simulink model "Matrix12"  (R2021a)
settings: Solver=VariableStepAuto  StartTime=0.0  StopTime=1  RelTol=1e-3
undefined symbols (not defined in the file): DiscIntNeverNeededParam
libraries: spsDiodeLib x18, spsIGBTLib x18, simulink x6, spsIGBTDiodeLib x6, spsSeriesRLCBranchLib x4, spsThreePhaseVIMeasurementLib x3, spsSaturableTransformerLib x3, spsabctoAlphaBetaZeroLib x2, spsAlphaBetaZerotoabcLib x1, pid_lib x1, spsSecondOrderFilterLib x1, spsThreePhaseSeriesRLCBranchLib x1
(part 1 of 2)
settings Model: SimulationMode=accelerator  Creator=HP  LastModifiedBy=HP

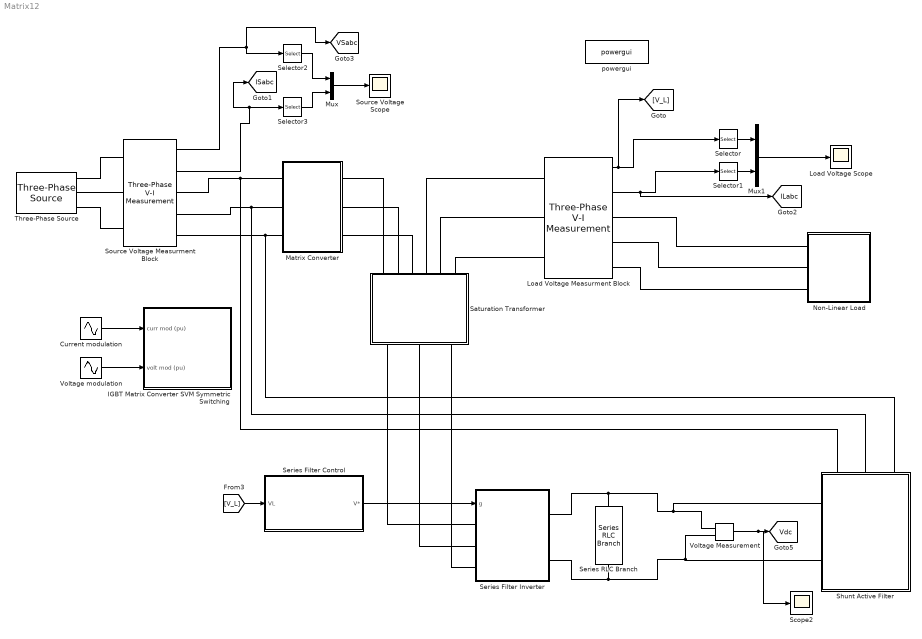
== system Matrix12 ==
  Current modulation : Sin  Amplitude=1*sqrt(2)/sqrt(3)  Frequency=2*pi*1000  Phase=[0 -2*pi/3 2*pi/3]  SampleTime=0
  IGBT Matrix Converter SVM Symmetric Switching : Subsystem
  Load Voltage Measurment Block : spsThreePhaseVIMeasurementLib/Three-Phase V-I Measurement  VoltageMeasurement=phase-to-phase  SetLabelV=off  LabelV=V_L  Vpu=off  VpuLL=off  CurrentMeasurement=yes  SetLabelI=off  LabelI=Iabc  Ipu=off  Pbase=100e6  Vbase=500e3  OutputType=Complex  PhasorSimulation=off  PSBequivalent=0
  Load Voltage Scope : Scope
  Matrix Converter : Subsystem
  Mux : Mux  Inputs=2
  Mux1 : Mux  Inputs=2
  Non-Linear Load : Subsystem
  Saturation Transformer : Subsystem
  Scope2 : Scope
  Selector{,1..3} (4 alike) : Selector  InputPortWidth=3  IndexOptions=Index vector (dialog)  Indices=1  OutputSizes=1
  Series Filter Inverter : Subsystem
      mask Display: fprintf('series\nfilter')
  Series Filter Control : Subsystem
      mask Display: fprintf('Series\nFilter')
  Series RLC Branch : spsSeriesRLCBranchLib/Series RLC Branch  LConnTagsString=__new0  RConnTagsString=__new0  BranchType=C  Resistance=1  Inductance=1e-3  SetiL0=off  InitialCurrent=0  Capacitance=10  Setx0=on  InitialVoltage=700  Measurements=None
  Shunt Active Filter : Subsystem
      settings: PortSchema="{\"entries\":[{\"content\":{\"sides\":[{\"content\":{\"connectorIds\":[]},\"type\":\"ConnectorPlacement.EquallySpacedRectSide\",\"uuid\":\"661bd002-34f2-471b-8915-a7d9af4edb84\"},{\"content\":{\"connectorIds\":[\"RConn1\",\"RConn2\"],\"side\":\"RIGHT\"},\"type\":\"ConnectorPlacement.EquallySpacedRectSide\",\"uuid\":\"4a3a3177-9c19-4181-9982-d76e774c7df0\"},{\"content\":{\"connectorIds\":[\"LConn1\",\"LConn2\",\"LConn3\"],\"side\":\"TOP\"},\"type\":\"ConnectorPlacement.EquallySpacedRectSide\",\"uuid\":\"acd6b456-b827-42fc-a7ca-c38254438ca2\"}]},\"type\":\"ConnectorPlacement.EquallySpacedConnector\",\"uuid\":\"b55db1d3-6588-49b1-b57b-fb04199798b7\"}],\"packageUris\":[\"http://schema.mathworks.com/mf0/Connector/R2020b\"],\"version\":\"1.0\"}"
  Source Voltage Measurment Block : spsThreePhaseVIMeasurementLib/Three-Phase V-I Measurement  VoltageMeasurement=phase-to-ground  SetLabelV=off  LabelV=Vabc  Vpu=off  VpuLL=off  CurrentMeasurement=yes  SetLabelI=off  LabelI=Iabc  Ipu=off  Pbase=100e6  Vbase=500e3  OutputType=Complex  PhasorSimulation=off  PSBequivalent=0
  Source Voltage Scope : Scope
  Three-Phase Source : spsThreePhaseSourceLib/Three-Phase Source  InternalConnection=Yg  VoltagePhases=on  Voltage=400  PhaseAngle=0  Voltage_phases=[400 400 400]/sqrt(3)  PhaseAngles_phases=[0 -120 +120]  Frequency=50  NonIdealSource=off  SpecifyImpedance=off  Resistance=0.8929  Inductance=16.58e-3  ShortCircuitLevel=100e6  BaseVoltage=25e3  XRratio=7  BusType=swing  Pref=10e3  Qref=0  Prefabc=[10e3, 10e3, 10e3]  Qrefabc=[0, 0, 0]  Qmin=-inf  Qmax=inf
  Voltage Measurement : spsVoltageMeasurementLib/Voltage Measurement  PhasorSimulation=off  OutputType=Complex  PSBequivalent=0
  Voltage modulation : Sin  Amplitude=1*sqrt(2)/sqrt(3)  Frequency=2*pi*1000  Phase=[0 -2*pi/3 2*pi/3]  SampleTime=0
  powergui : spspowerguiLib/powergui  SimulationMode=Discrete  SampleTime=2e-6  frequency=50  Iterations=50  frequencyindice=50  Pbase=100e6  ErrMax=1e-4  UnitsV=kV  UnitsW=MW  buscounter=0  FunctionMessages=off  echomessages=off  EnableUseOfTLC=off  CurrentSourceSwitches=off  DisableSnubberDevices=off  DisableRonSwitches=off  DisableVfSwitches=off  DisplayEquations=off  AutomaticDiscreteSolvers=off  SolverType=Tustin/Backward Euler (TBE)  Interpol=off  ExternalGateDelay=off  methode=off  Ts=100  x0status=blocks  SPID=off  SwTol=0  HookPort=off  NonlinearTolerance=1e-4  nMaxIteration=100  ContinueOnMaxIteration=off  RestoreLinks=warning  ResistiveCurrentMeasurement=off  Frange=[0:2:500]  Ylog=off  Xlog=on  ShowGrid=off  save=off  variable=ZData  structure=Vs  ZoomFFT=on  StartTime=1/60  cycles=1  DisplayStyle=1  fundamental=60  FreqAxis=on  MaxFrequency=10000  frequencyindicesteady=1  RmsSteady=1  display=off
  tag scope: ILabc=global, ISabc=global, VSabc=global, Vdc=global
  wires:
  [V_L] -> Series Filter Control/1(VL)
  Mux/1 -> Source Voltage Scope/1
  Selector1/1 -> Mux1/2
  Selector/1 -> Mux1/1
  Load Voltage Measurment Block/1 -> [V_L], Selector/1
  Selector3/1 -> Mux/2
  Source Voltage Measurment Block/1 -> Selector2/1, [VSabc]
  Series Filter Control/1(V*) -> Series Filter Inverter/1(g)
  Source Voltage Measurment Block/2 -> [ISabc], Selector3/1
  Voltage modulation/1 -> IGBT Matrix Converter SVM Symmetric Switching/2(volt mod (pu))
  Load Voltage Measurment Block/2 -> [ILabc], Selector1/1
  Mux1/1 -> Load Voltage Scope/1
  Current modulation/1 -> IGBT Matrix Converter SVM Symmetric Switching/1(curr mod (pu))
  Selector2/1 -> Mux/1
  Voltage Measurement/1 -> Scope2/1, [Vdc]
  connections:
  Series Filter Inverter/LConn3 -- Saturation Transformer/LConn3
  Series Filter Inverter/LConn1 -- Saturation Transformer/LConn1
  Saturation Transformer/RConn3 -- Matrix Converter/RConn3
  Saturation Transformer/RConn4 -- Load Voltage Measurment Block/LConn1
  Source Voltage Measurment Block/RConn2 -- Matrix Converter/LConn2 -- Shunt Active Filter/LConn2
  Saturation Transformer/RConn5 -- Load Voltage Measurment Block/LConn2
  Series Filter Inverter/LConn2 -- Saturation Transformer/LConn2
  Three-Phase Source/RConn1 -- Source Voltage Measurment Block/LConn1
  Source Voltage Measurment Block/RConn3 -- Shunt Active Filter/LConn1 -- Matrix Converter/LConn3
  Three-Phase Source/RConn2 -- Source Voltage Measurment Block/LConn2
  Saturation Transformer/RConn1 -- Matrix Converter/RConn1
  Three-Phase Source/RConn3 -- Source Voltage Measurment Block/LConn3
  Saturation Transformer/RConn2 -- Matrix Converter/RConn2
  Saturation Transformer/RConn6 -- Load Voltage Measurment Block/LConn3
  Matrix Converter/LConn1 -- Shunt Active Filter/LConn3 -- Source Voltage Measurment Block/RConn1
  Voltage Measurement/LConn1 -- Series RLC Branch/LConn1 -- Series Filter Inverter/RConn1 -- Shunt Active Filter/RConn1
  Shunt Active Filter/RConn2 -- Series RLC Branch/RConn1 -- Series Filter Inverter/RConn2 -- Voltage Measurement/LConn2
  Load Voltage Measurment Block/RConn1 -- Non-Linear Load/LConn1
  Load Voltage Measurment Block/RConn2 -- Non-Linear Load/LConn2
  Load Voltage Measurment Block/RConn3 -- Non-Linear Load/LConn3

== system Matrix12/IGBT Matrix Converter SVM Symmetric Switching ==
  curr mod (pu) : Inport
  volt mod (pu) : Inport  Port=2
  SVM Inversion symmetric sequence : Subsystem  mask{switching_freq=1000}
      mask prompts: switching_freq "switching frequency (Hz)"
  SVM Rectification symmetric sequence : Subsystem  mask{switching_freq=1000}
      mask prompts: switching_freq "switching frequency (Hz)"
  matrix converter switching : Subsystem
  wires:
  SVM Inversion symmetric sequence/1(g) -> matrix converter switching/2(gI)
  SVM Rectification symmetric sequence/1(g) -> matrix converter switching/1(gR)
  curr mod (pu)/1 -> SVM Rectification symmetric sequence/1(mod (pu))
  volt mod (pu)/1 -> SVM Inversion symmetric sequence/1(mod (pu))

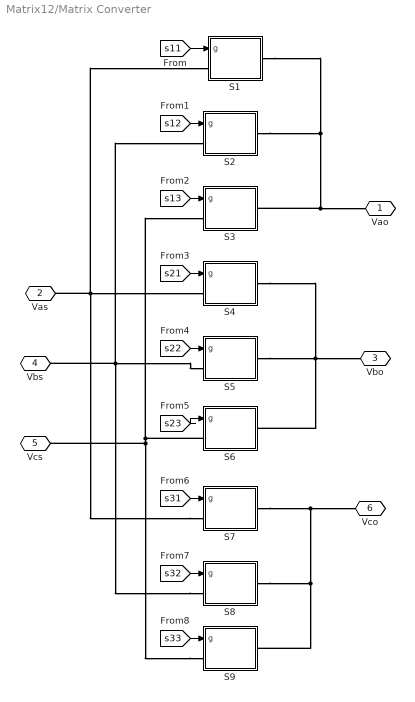
== system Matrix12/Matrix Converter ==
  S1 : Subsystem
  S2 : Subsystem
  S3 : Subsystem
  S4 : Subsystem
  S5 : Subsystem
  S6 : Subsystem
  S7 : Subsystem
  S8 : Subsystem
  S9 : Subsystem
  Vao : PMIOPort  Side=Right
  Vas : PMIOPort  Port=2  Side=Left
  Vbo : PMIOPort  Port=3  Side=Right
  Vbs : PMIOPort  Port=4  Side=Left
  Vcs : PMIOPort  Port=5  Side=Left
  Vco : PMIOPort  Port=6  Side=Right
  wires:
  [s12] -> S2/1(g)
  [s13] -> S3/1(g)
  [s32] -> S8/1(g)
  [s11] -> S1/1(g)
  [s33] -> S9/1(g)
  [s31] -> S7/1(g)
  [s23] -> S6/1(g)
  [s22] -> S5/1(g)
  [s21] -> S4/1(g)
  connections:
  S3/RConn1 -- S1/RConn1 -- S2/RConn1 -- Vao/RConn1
  S7/LConn1 -- S1/LConn1 -- S4/LConn1 -- Vas/RConn1
  S6/RConn1 -- S4/RConn1 -- S5/RConn1 -- Vbo/RConn1
  S8/LConn1 -- S2/LConn1 -- S5/LConn1 -- Vbs/RConn1
  S9/RConn1 -- S8/RConn1 -- S7/RConn1 -- Vco/RConn1
  S9/LConn1 -- S3/LConn1 -- S6/LConn1 -- Vcs/RConn1

== system Matrix12/Non-Linear Load ==
  Series RLC Branch : spsSeriesRLCBranchLib/Series RLC Branch  LConnTagsString=__new0  RConnTagsString=__new0  BranchType=RL  Resistance=10  Inductance=1e-6  SetiL0=off  InitialCurrent=0  Capacitance=1e-6  Setx0=off  InitialVoltage=0  Measurements=None
  Series RLC Branch1 : spsSeriesRLCBranchLib/Series RLC Branch  LConnTagsString=__new0  RConnTagsString=__new0  BranchType=RL  Resistance=10  Inductance=1e-6  SetiL0=off  InitialCurrent=0  Capacitance=1e-6  Setx0=off  InitialVoltage=0  Measurements=None
  Series RLC Branch2 : spsSeriesRLCBranchLib/Series RLC Branch  LConnTagsString=__new0  RConnTagsString=__new0  BranchType=RL  Resistance=10  Inductance=1e-6  SetiL0=off  InitialCurrent=0  Capacitance=1e-6  Setx0=off  InitialVoltage=0  Measurements=None
  a : PMIOPort  Side=Left
  b : PMIOPort  Port=2  Side=Left
  c : PMIOPort  Port=3  Side=Left
  connections:
  a/RConn1 -- Series RLC Branch/LConn1
  Series RLC Branch/RConn1 -- Series RLC Branch1/RConn1 -- Series RLC Branch2/RConn1
  b/RConn1 -- Series RLC Branch1/LConn1
  c/RConn1 -- Series RLC Branch2/LConn1

== system Matrix12/Saturation Transformer ==
  Tc_a : spsSaturableTransformerLib/Saturable Transformer  ThreeWindings=off  Hysteresis=off  DataFile='hysteresis.mat'  Measurements=None  UNITS=pu  NominalPower=[4000 50]  Winding1="[400  0.02  0.02 ]"  Winding2="[400  0.02  0.02]"  Winding3="[ 315e3  0.002  0.08 ]"  Saturation=[ 0 0 ;1.016 9.043]*1e-3  CoreLoss=[117 0]  BreakLoop=off  DiscreteSolver=Trapezoidal iterative  DataType=off  InitialFlux=0  TransfoNumber=1
      settings: SourceProductBaseCode=PS
  Tc_b : spsSaturableTransformerLib/Saturable Transformer  ThreeWindings=off  Hysteresis=off  DataFile='hysteresis.mat'  Measurements=None  UNITS=pu  NominalPower=[4000 50]  Winding1="[400  0.02  0.02 ]"  Winding2="[400  0.02  0.02]"  Winding3="[ 315e3  0.002  0.08 ]"  Saturation=[ 0 0 ;1.016 9.043]*1e-3  CoreLoss=[117 0]  BreakLoop=off  DiscreteSolver=Trapezoidal iterative  DataType=off  InitialFlux=0  TransfoNumber=1
      settings: SourceProductBaseCode=PS
  Tc_c : spsSaturableTransformerLib/Saturable Transformer  ThreeWindings=off  Hysteresis=off  DataFile='hysteresis.mat'  Measurements=None  UNITS=pu  NominalPower=[4000 50]  Winding1="[400  0.02  0.02 ]"  Winding2="[400  0.02  0.02]"  Winding3="[ 315e3  0.002  0.08 ]"  Saturation=[ 0 0 ;1.016 9.043]*1e-3  CoreLoss=[117 0]  BreakLoop=off  DiscreteSolver=Trapezoidal iterative  DataType=off  InitialFlux=0  TransfoNumber=1
      settings: SourceProductBaseCode=PS
  A : PMIOPort  Side=Left
  B : PMIOPort  Port=2  Side=Left
  C : PMIOPort  Port=3  Side=Left
  Vain : PMIOPort  Port=4  Side=Right
  Vbin : PMIOPort  Port=5  Side=Right
  Vcin : PMIOPort  Port=6  Side=Right
  Vao : PMIOPort  Port=7  Side=Right
  Vbo : PMIOPort  Port=8  Side=Right
  Vco : PMIOPort  Port=9  Side=Right
  connections:
  Tc_c/LConn2 -- C/RConn1
  Tc_a/RConn2 -- Vao/RConn1
  Vcin/RConn1 -- Tc_c/RConn1
  Tc_a/LConn1 -- Tc_c/LConn1 -- Tc_b/LConn1
  Tc_b/LConn2 -- B/RConn1
  Vain/RConn1 -- Tc_a/RConn1
  Tc_c/RConn2 -- Vco/RConn1
  Vbin/RConn1 -- Tc_b/RConn1
  Tc_b/RConn2 -- Vbo/RConn1
  Tc_a/LConn2 -- A/RConn1

== system Matrix12/Series Filter Inverter ==
  g : Inport
  Demux : Demux  Outputs=3
      settings: DisplayOption=none
  Logical Operator : Logic  Operator=NOT  AllPortsSameDT=off  OutDataTypeStr=boolean
  Logical Operator1 : Logic  Operator=NOT  AllPortsSameDT=off  OutDataTypeStr=boolean
  Logical Operator2 : Logic  Operator=NOT  AllPortsSameDT=off  OutDataTypeStr=boolean
  s{1..6} (6 alike) : spsIGBTDiodeLib/IGBT//Diode  Ron=1e-3  Rs=1e5  Cs=inf  Measurements=off
  + : PMIOPort  Side=Right
  - : PMIOPort  Port=2  Side=Right
  A : PMIOPort  Port=3  Side=Left
  B : PMIOPort  Port=4  Side=Left
  C : PMIOPort  Port=5  Side=Left
  wires:
  Demux/2 -> s3/1, Logical Operator1/1
  Demux/1 -> s1/1, Logical Operator/1
  Logical Operator/1 -> s2/1
  Logical Operator1/1 -> s4/1
  Logical Operator2/1 -> s6/1
  Demux/3 -> Logical Operator2/1, s5/1
  g/1 -> Demux/1
  connections:
  +/RConn1 -- s5/LConn1 -- s1/LConn1 -- s3/LConn1
  A/RConn1 -- s2/LConn1 -- s1/RConn1
  -/RConn1 -- s6/RConn1 -- s4/RConn1 -- s2/RConn1
  B/RConn1 -- s4/LConn1 -- s3/RConn1
  C/RConn1 -- s5/RConn1 -- s6/LConn1

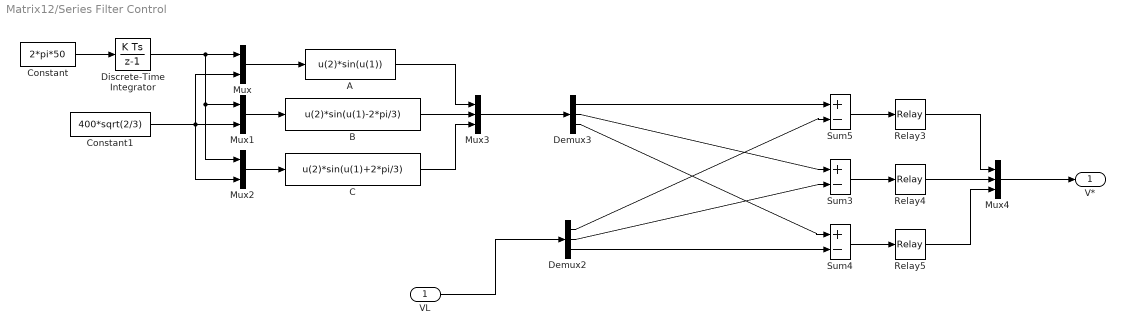
== system Matrix12/Series Filter Control ==
  VL : Inport
  A : Fcn  Expr=u(2)*sin(u(1))
  B : Fcn  Expr=u(2)*sin(u(1)-2*pi/3)
  C : Fcn  Expr=u(2)*sin(u(1)+2*pi/3)
  Constant : Constant  Value=2*pi*50
  Constant1 : Constant  Value=400*sqrt(2/3)
  Demux2 : Demux  Outputs=3
  Demux3 : Demux  Outputs=3
  Discrete-Time Integrator : DiscreteIntegrator  SampleTime=2e-6  ICPrevOutput=DiscIntNeverNeededParam  ICPrevScaledInput=DiscIntNeverNeededParam
  Mux : Mux  Inputs=2
  Mux1 : Mux  Inputs=2
  Mux2 : Mux  Inputs=2
  Mux3 : Mux  Inputs=3
  Mux4 : Mux  Inputs=3
  Relay3 : Relay  OnSwitchValue=1  OffSwitchValue=-1
  Relay4 : Relay  OnSwitchValue=1  OffSwitchValue=-1
  Relay5 : Relay  OnSwitchValue=1  OffSwitchValue=-1
  Sum3 : Sum  Inputs=+-
  Sum4 : Sum  Inputs=+-
  Sum5 : Sum  Inputs=+-
  V* : Outport
  wires:
  Constant/1 -> Discrete-Time Integrator/1
  Discrete-Time Integrator/1 -> Mux/1, Mux2/1, Mux1/1
  Constant1/1 -> Mux1/2, Mux2/2, Mux/2
  Mux/1 -> A/1
  Mux1/1 -> B/1
  Mux2/1 -> C/1
  A/1 -> Mux3/1
  B/1 -> Mux3/2
  C/1 -> Mux3/3
  Sum5/1 -> Relay3/1
  Sum3/1 -> Relay4/1
  Sum4/1 -> Relay5/1
  Relay3/1 -> Mux4/1
  Relay4/1 -> Mux4/2
  Relay5/1 -> Mux4/3
  Mux4/1 -> V*/1
  VL/1 -> Demux2/1
  Demux3/1 -> Sum5/1
  Demux2/3 -> Sum4/2
  Demux2/1 -> Sum5/2
  Demux3/3 -> Sum4/1
  Demux2/2 -> Sum3/2
  Demux3/2 -> Sum3/1
  Mux3/1 -> Demux3/1

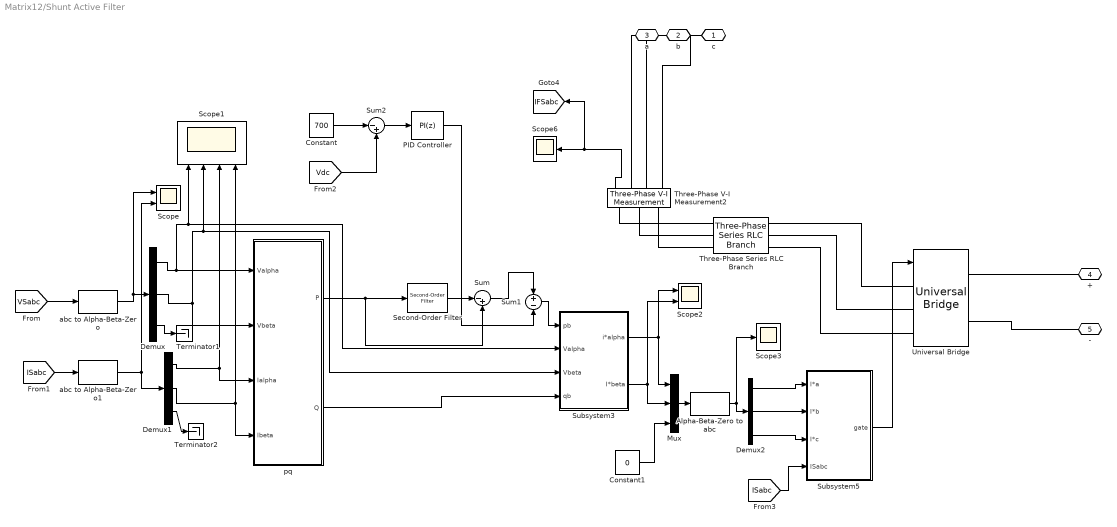
== system Matrix12/Shunt Active Filter ==
  Alpha-Beta-Zero to abc : spsAlphaBetaZerotoabcLib/Alpha-Beta-Zero to abc
      settings: SourceProductBaseCode=PS
  Constant : Constant  Value=700
  Constant1 : Constant  Value=0
  Demux : Demux  Outputs=3
  Demux1 : Demux  Outputs=3
  Demux2 : Demux  Outputs=3
  Mux : Mux  Inputs=3
  PID Controller : pid_lib/PID Controller  Controller=PI  Form=Parallel  TimeDomain=Discrete-time  UseExternalTs=off  SampleTime=-1  IntegratorMethod=Forward Euler  FilterMethod=Forward Euler  ControllerParametersSource=internal  P=0.01  I=1  D=0  UseFilter=on  N=100  TunerSelectOption=Transfer Function Based (PID Tuner App)  InitialConditionSource=internal  InitialConditionForIntegrator=0  InitialConditionForFilter=0  DifferentiatorICPrevScaledInput=0  ExternalReset=none  TrackingMode=off  Kt=1  LimitOutput=off  SatLimitsSource=internal  UpperSaturationLimit=inf  LowerSaturationLimit=-inf  LinearizeAsGain=on  AntiWindupMode=none  Kb=1  POutMin=[]  POutMax=[]  IOutMin=[]  IOutMax=[]  DOutMin=[]  DOutMax=[]  NOutMin=[]  NOutMax=[]  SumOutMin=[]  SumOutMax=[]  SaturationOutMin=[]  SaturationOutMax=[]  PParamMin=[]  PParamMax=[]  IParamMin=[]  IParamMax=[]  DParamMin=[]  DParamMax=[]  NParamMin=[]  NParamMax=[]  KbParamMin=[]  KbParamMax=[]  KtParamMin=[]  KtParamMax=[]  KbOutMin=[]  KbOutMax=[]  KtOutMin=[]  KtOutMax=[]  IntegratorOutMin=[]  IntegratorOutMax=[]  FilterOutMin=[]  FilterOutMax=[]  SumI1OutMin=[]  SumI1OutMax=[]  SumI2OutMin=[]  SumI2OutMax=[]  SumI3OutMin=[]  SumI3OutMax=[]  SumI4OutMin=[]  SumI4OutMax=[]  SumDOutMin=[]  SumDOutMax=[]  DifferentiatorOutMin=[]  DifferentiatorOutMax=[]  FilterDiffOutCoefMin=[]  FilterDiffOutCoefMax=[]  ReciprocalOutMin=[]  ReciprocalOutMax=[]  SumDenOutMin=[]  SumDenOutMax=[]  SumNumOutMin=[]  SumNumOutMax=[]  DivideOutMin=[]  DivideOutMax=[]  UdiffTsProdOutMin=[]  UdiffTsProdOutMax=[]  NTsProdOutMin=[]  NTsProdOutMax=[]  UintegralTsProdOutMin=[]  UintegralTsProdOutMax=[]  UngainTsProdOutMin=[]  UngainTsProdOutMax=[]  IntegratorContinuousStateAttributes=''  IntegratorStateMustResolveToSignalObject=off  IntegratorRTWStateStorageClass=Auto  FilterContinuousStateAttributes=''  FilterStateMustResolveToSignalObject=off  FilterRTWStateStorageClass=Auto  ParallelPVariant=InternalParameters  IdealPVariant=Disabled  IVariant=InternalParameters  DVariant=Disabled  IntegratorVariant=Discrete  SatVariant=Disabled  AWVariant=Passthrough  PCopyVariant=Disabled  TRVariant=Disabled  FdbkBlocksVariant=Forward  IdealPFdbkVariant=Disabled  SatFdbkVariant=Disabled  DerivativeFilterVariant=Disabled  NVariant=Disabled  NCopyVariant=Disabled_SignalSpec  FilterICVariant=Disabled  IntegratorICVariant=InternalICs  ExternalResetVariant=Disabled  TRSumVariant=Passthrough  SumFdbkVariant=Disabled  SumVariant=Sum_PI  TsampFilterVariant=InternalTs  TsampNgainVariant=Passthrough  TsampIntegralVariant=Passthrough  ExternalSaturationOutDataTypeStr=Inherit: Same as second input
  Scope : Scope  NumInputPorts=2
  Scope1 : Scope  NumInputPorts=4
  Scope2 : Scope  NumInputPorts=2
  Scope3 : Scope
  Scope6 : Scope
  Second-Order Filter : spsSecondOrderFilterLib/Second-Order Filter  FilterType=Lowpass  Fo=40000  Zeta=0.707  Ts=0  Initialize=on  Vac_Init="[0,  0,  50]"  Vdc_Init=0  PlotResponse=off  FreqRange=[0, 500, 1]
      settings: SourceProductBaseCode=PS
  Subsystem3 : Subsystem
  Subsystem5 : Subsystem
  Sum : Sum  Inputs=|-+
  Sum1 : Sum  Inputs=+|-
  Sum2 : Sum  Inputs=|-+
  Terminator1 : Terminator
  Terminator2 : Terminator
  Three-Phase Series RLC Branch : spsThreePhaseSeriesRLCBranchLib/Three-Phase Series RLC Branch  LConnTagsString=A|B|C  RConnTagsString=A|B|C  BranchType=L  Resistance=1  Inductance=2e-3  Capacitance=1e-6  Measurements=None
  Three-Phase V-I Measurement2 : spsThreePhaseVIMeasurementLib/Three-Phase V-I Measurement  VoltageMeasurement=no  SetLabelV=off  LabelV=Vabc  Vpu=off  VpuLL=off  CurrentMeasurement=yes  SetLabelI=off  LabelI=Iabc  Ipu=off  Pbase=100e6  Vbase=500e3  OutputType=Complex  PhasorSimulation=off  PSBequivalent=0
  Universal Bridge : spsUniversalBridgeLib/Universal Bridge  Arms=3  SnubberResistance=1e5  SnubberCapacitance=inf  Device=MOSFET / Diodes  Ron=1e-3  Lon=0  ForwardVoltages="[  0  0  ]"  ForwardVoltage=0  GTOparameters=[ 10e-6 , 20e-6 ]  IGBTparameters=[ 1e-6 , 2e-6 ]  Measurements=None  Measurements_2=None  converterType=Rectifier
  abc to Alpha-Beta-Zero : spsabctoAlphaBetaZeroLib/abc to Alpha-Beta-Zero
      settings: SourceProductBaseCode=PS
  abc to Alpha-Beta-Zero1 : spsabctoAlphaBetaZeroLib/abc to Alpha-Beta-Zero
      settings: SourceProductBaseCode=PS
  pq : Subsystem
  c : PMIOPort  Side=Left
  b : PMIOPort  Port=2  Side=Left
  a : PMIOPort  Port=3  Side=Left
  + : PMIOPort  Port=4  Side=Right
  - : PMIOPort  Port=5  Side=Right
  tag scope: IFSabc=global
  wires:
  Subsystem3/1(i*alpha) -> Mux/1, Scope2/1
  Demux1/1 -> pq/3(Ialpha), Scope1/3
  Demux1/2 -> pq/4(Ibeta), Scope1/4
  Alpha-Beta-Zero to abc/1 -> Demux2/1, Scope3/1
  Three-Phase V-I Measurement2/1 -> Scope6/1, [IFSabc]
  Demux2/1 -> Subsystem5/1(I*a)
  Demux1/3 -> Terminator2/1
  Demux/1 -> Subsystem3/2(Valpha), Scope1/1, pq/1(Valpha)
  pq/2(Q) -> Subsystem3/4(qb)
  Sum2/1 -> PID Controller/1
  pq/1(P) -> Second-Order Filter/1, Sum/2
  [Vdc] -> Sum2/2
  Demux/2 -> pq/2(Vbeta), Subsystem3/3("Vbeta "), Scope1/2
  [ISabc] -> Subsystem5/4(ISabc)
  Demux/3 -> Terminator1/1
  abc to Alpha-Beta-Zero1/1 -> Scope/2, Demux1/1
  Demux2/2 -> Subsystem5/2(I*b)
  Subsystem5/1("gate ") -> Universal Bridge/1
  Sum/1 -> Sum1/1
  PID Controller/1 -> Sum1/2
  Sum1/1 -> Subsystem3/1(pb)
  Constant/1 -> Sum2/1
  Subsystem3/2("I*beta ") -> Mux/2, Scope2/2
  Second-Order Filter/1 -> Sum/1
  Demux2/3 -> Subsystem5/3(I*c)
  Mux/1 -> Alpha-Beta-Zero to abc/1
  [ISabc] -> abc to Alpha-Beta-Zero1/1
  abc to Alpha-Beta-Zero/1 -> Scope/1, Demux/1
  Constant1/1 -> Mux/3
  [VSabc] -> abc to Alpha-Beta-Zero/1
  connections:
  Three-Phase V-I Measurement2/RConn3 -- c/RConn1
  Three-Phase V-I Measurement2/LConn3 -- Three-Phase Series RLC Branch/LConn3
  Three-Phase Series RLC Branch/RConn1 -- Universal Bridge/LConn1
  Three-Phase Series RLC Branch/RConn2 -- Universal Bridge/LConn2
  Three-Phase Series RLC Branch/RConn3 -- Universal Bridge/LConn3
  +/RConn1 -- Universal Bridge/RConn1
  Three-Phase V-I Measurement2/LConn1 -- Three-Phase Series RLC Branch/LConn1
  Three-Phase V-I Measurement2/LConn2 -- Three-Phase Series RLC Branch/LConn2
  Universal Bridge/RConn2 -- -/RConn1
  Three-Phase V-I Measurement2/RConn2 -- b/RConn1
  Three-Phase V-I Measurement2/RConn1 -- a/RConn1

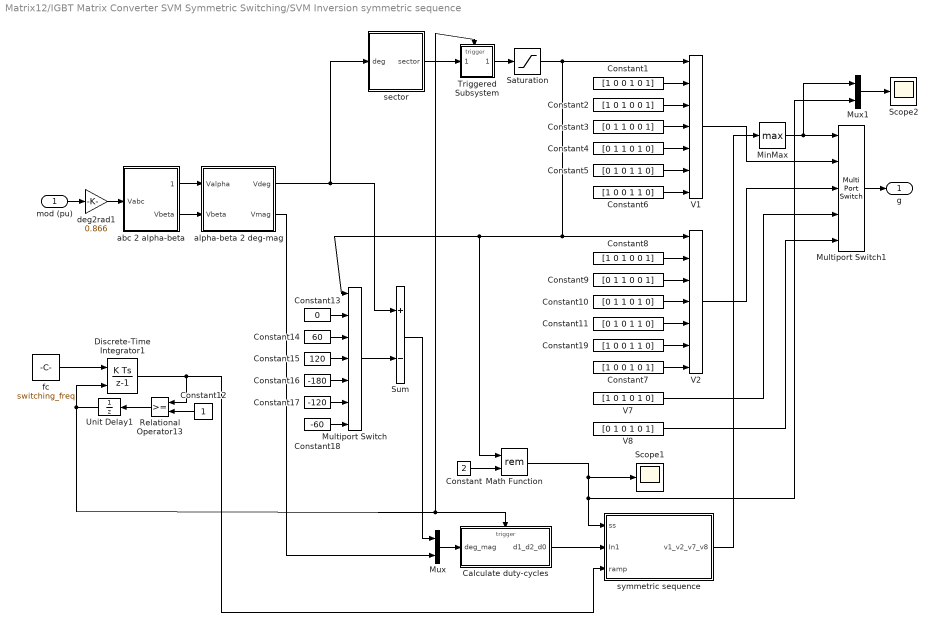
== system Matrix12/IGBT Matrix Converter SVM Symmetric Switching/SVM Inversion symmetric sequence ==
  mod (pu) : Inport
  Calculate duty-cycles : Subsystem  TreatAsAtomicUnit=on
  Constant : Constant  Value=2
  Constant1 : Constant  Value=[1 0 0 1 0 1]
  Constant10 : Constant  Value=[0 1 1 0 1 0]
  Constant11 : Constant  Value=[0 1 0 1 1 0]
  Constant12 : Constant
  Constant13 : Constant  Value=0
  Constant14 : Constant  Value=60
  Constant15 : Constant  Value=120
  Constant16 : Constant  Value=-180
  Constant17 : Constant  Value=-120
  Constant18 : Constant  Value=-60
  Constant19 : Constant  Value=[1 0 0 1 1 0]
  Constant2 : Constant  Value=[1 0 1 0 0 1]
  Constant3 : Constant  Value=[0 1 1 0 0 1]
  Constant4 : Constant  Value=[0 1 1 0 1 0]
  Constant5 : Constant  Value=[0 1 0 1 1 0]
  Constant6 : Constant  Value=[1 0 0 1 1 0]
  Constant7 : Constant  Value=[1 0 0 1 0 1]
  Constant8 : Constant  Value=[1 0 1 0 0 1]
  Constant9 : Constant  Value=[0 1 1 0 0 1]
  Discrete-Time Integrator1 : DiscreteIntegrator  ExternalReset=rising  SampleTime=2e-6  ICPrevOutput=DiscIntNeverNeededParam  ICPrevScaledInput=DiscIntNeverNeededParam
  Math Function : Math  Operator=rem  SignedPower=on  SaturateOnIntegerOverflow=on
  MinMax : MinMax  Function=max
  Multiport Switch : MultiPortSwitch  Inputs=6
  Multiport Switch1 : MultiPortSwitch  Inputs=4
  Mux : Mux  Inputs=2
  Mux1 : Mux  Inputs=2
  Relational Operator13 : RelationalOperator  RndMeth=Nearest  InputSameDT=on
  Saturation : Saturate  UpperLimit=6  LowerLimit=1
  Scope1 : Scope
  Scope2 : Scope
  Sum : Sum  Inputs=+-
  Triggered Subsystem : Subsystem  TreatAsAtomicUnit=on
  Unit Delay1 : UnitDelay  SampleTime=2e-6  HasFrameUpgradeWarning=on
  V1 : MultiPortSwitch  Inputs=6
  V2 : MultiPortSwitch  Inputs=6
  V7 : Constant  Value=[1 0 1 0 1 0]
  V8 : Constant  Value=[0 1 0 1 0 1]
  abc 2 alpha-beta : Subsystem
  alpha-beta 2 deg-mag : Subsystem
  deg2rad1 : Gain  Gain=0.866
  fc : Constant  Value=switching_freq
  sector : Subsystem
  symmetric sequence : Subsystem
  g : Outport  VectorParamsAs1DForOutWhenUnconnected=off
  wires:
  Mux1/1 -> Scope2/1
  Math Function/1 -> Mux1/2, symmetric sequence/1(ss), Scope1/1
  symmetric sequence/1(v1_v2_v7_v8) -> MinMax/1
  Constant/1 -> Math Function/2
  deg2rad1/1 -> abc 2 alpha-beta/1(Vabc)
  Triggered Subsystem/1(Out1) -> Saturation/1
  sector/1(sector) -> Triggered Subsystem/1(In1)
  Saturation/1 -> V1/1, Math Function/1, Multiport Switch/1, V2/1
  Unit Delay1/1 -> Calculate duty-cycles/Trigger, Triggered Subsystem/Trigger, Discrete-Time Integrator1/2
  Multiport Switch1/1 -> g/1
  MinMax/1 -> Mux1/1, Multiport Switch1/1
  V8/1 -> Multiport Switch1/5
  V7/1 -> Multiport Switch1/4
  V2/1 -> Multiport Switch1/3
  V1/1 -> Multiport Switch1/2
  Constant7/1 -> V2/7
  Constant6/1 -> V1/7
  Constant2/1 -> V1/3
  Constant19/1 -> V2/6
  Constant11/1 -> V2/5
  Constant10/1 -> V2/4
  Constant9/1 -> V2/3
  Constant8/1 -> V2/2
  Constant5/1 -> V1/6
  Constant4/1 -> V1/5
  Constant3/1 -> V1/4
  Constant1/1 -> V1/2
  Sum/1 -> Mux/1
  Multiport Switch/1 -> Sum/2
  Constant18/1 -> Multiport Switch/7
  Constant17/1 -> Multiport Switch/6
  Constant16/1 -> Multiport Switch/5
  Constant15/1 -> Multiport Switch/4
  Constant14/1 -> Multiport Switch/3
  Constant13/1 -> Multiport Switch/2
  Calculate duty-cycles/1(d1_d2_d0) -> symmetric sequence/2(In1)
  abc 2 alpha-beta/2(Vbeta) -> alpha-beta 2 deg-mag/2(Vbeta)
  abc 2 alpha-beta/1(Valpha) -> alpha-beta 2 deg-mag/1(Valpha)
  Mux/1 -> Calculate duty-cycles/1(deg_mag)
  fc/1 -> Discrete-Time Integrator1/1
  Discrete-Time Integrator1/1 -> symmetric sequence/3(ramp), Relational Operator13/1
  Constant12/1 -> Relational Operator13/2
  Relational Operator13/1 -> Unit Delay1/1
  alpha-beta 2 deg-mag/2(Vmag) -> Mux/2
  alpha-beta 2 deg-mag/1(Vdeg) -> sector/1(deg), Sum/1
  mod (pu)/1 -> deg2rad1/1

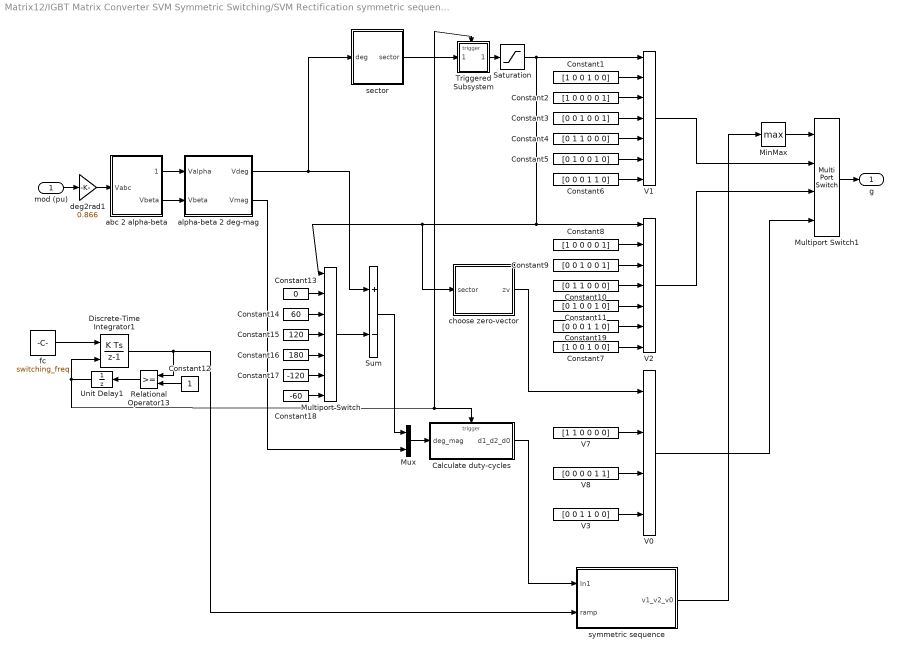
== system Matrix12/IGBT Matrix Converter SVM Symmetric Switching/SVM Rectification symmetric sequence ==
  mod (pu) : Inport
  Calculate duty-cycles : Subsystem  TreatAsAtomicUnit=on
  Constant1 : Constant  Value=[1 0 0 1 0 0]
  Constant10 : Constant  Value=[0 1 1 0 0 0]
  Constant11 : Constant  Value=[0 1 0 0 1 0]
  Constant12 : Constant
  Constant13 : Constant  Value=0
  Constant14 : Constant  Value=60
  Constant15 : Constant  Value=120
  Constant16 : Constant  Value=180
  Constant17 : Constant  Value=-120
  Constant18 : Constant  Value=-60
  Constant19 : Constant  Value=[0 0 0 1 1 0]
  Constant2 : Constant  Value=[1 0 0 0 0 1]
  Constant3 : Constant  Value=[0 0 1 0 0 1]
  Constant4 : Constant  Value=[0 1 1 0 0 0]
  Constant5 : Constant  Value=[0 1 0 0 1 0]
  Constant6 : Constant  Value=[0 0 0 1 1 0]
  Constant7 : Constant  Value=[1 0 0 1 0 0]
  Constant8 : Constant  Value=[1 0 0 0 0 1]
  Constant9 : Constant  Value=[0 0 1 0 0 1]
  Discrete-Time Integrator1 : DiscreteIntegrator  ExternalReset=rising  SampleTime=2e-6  ICPrevOutput=DiscIntNeverNeededParam  ICPrevScaledInput=DiscIntNeverNeededParam
  MinMax : MinMax  Function=max
  Multiport Switch : MultiPortSwitch  Inputs=6
  Multiport Switch1 : MultiPortSwitch
  Mux : Mux  Inputs=2
  Relational Operator13 : RelationalOperator  RndMeth=Nearest  InputSameDT=on
  Saturation : Saturate  UpperLimit=6  LowerLimit=1
  Sum : Sum  Inputs=+-
  Triggered Subsystem : Subsystem  TreatAsAtomicUnit=on
  Unit Delay1 : UnitDelay  SampleTime=2e-6  HasFrameUpgradeWarning=on
  V0 : MultiPortSwitch
  V1 : MultiPortSwitch  Inputs=6
  V2 : MultiPortSwitch  Inputs=6
  V3 : Constant  Value=[0 0 1 1 0 0]
  V7 : Constant  Value=[1 1 0 0 0 0]
  V8 : Constant  Value=[0 0 0 0 1 1]
  abc 2 alpha-beta : Subsystem
  alpha-beta 2 deg-mag : Subsystem
  choose zero-vector : Subsystem
  deg2rad1 : Gain  Gain=0.866
  fc : Constant  Value=switching_freq
  sector : Subsystem
  symmetric sequence : Subsystem
  g : Outport  VectorParamsAs1DForOutWhenUnconnected=off
  wires:
  deg2rad1/1 -> abc 2 alpha-beta/1(Vabc)
  Saturation/1 -> V1/1, V2/1, Multiport Switch/1, choose zero-vector/1(sector)
  Triggered Subsystem/1(Out1) -> Saturation/1
  sector/1(sector) -> Triggered Subsystem/1(In1)
  MinMax/1 -> Multiport Switch1/1
  Unit Delay1/1 -> Discrete-Time Integrator1/2, Calculate duty-cycles/Trigger, Triggered Subsystem/Trigger
  Multiport Switch1/1 -> g/1
  symmetric sequence/1(v1_v2_v0) -> MinMax/1
  V2/1 -> Multiport Switch1/3
  V1/1 -> Multiport Switch1/2
  Constant7/1 -> V2/7
  Constant6/1 -> V1/7
  Constant2/1 -> V1/3
  Constant19/1 -> V2/6
  Constant11/1 -> V2/5
  Constant10/1 -> V2/4
  Constant9/1 -> V2/3
  Constant8/1 -> V2/2
  Constant5/1 -> V1/6
  Constant4/1 -> V1/5
  Constant3/1 -> V1/4
  Constant1/1 -> V1/2
  Sum/1 -> Mux/1
  Multiport Switch/1 -> Sum/2
  Constant18/1 -> Multiport Switch/7
  Constant17/1 -> Multiport Switch/6
  Constant16/1 -> Multiport Switch/5
  Constant15/1 -> Multiport Switch/4
  Constant14/1 -> Multiport Switch/3
  Constant13/1 -> Multiport Switch/2
  Calculate duty-cycles/1(d1_d2_d0) -> symmetric sequence/1(In1)
  abc 2 alpha-beta/2(Vbeta) -> alpha-beta 2 deg-mag/2(Vbeta)
  abc 2 alpha-beta/1(Valpha) -> alpha-beta 2 deg-mag/1(Valpha)
  Mux/1 -> Calculate duty-cycles/1(deg_mag)
  fc/1 -> Discrete-Time Integrator1/1
  Discrete-Time Integrator1/1 -> Relational Operator13/1, symmetric sequence/2(ramp)
  Constant12/1 -> Relational Operator13/2
  Relational Operator13/1 -> Unit Delay1/1
  alpha-beta 2 deg-mag/2(Vmag) -> Mux/2
  alpha-beta 2 deg-mag/1(Vdeg) -> sector/1(deg), Sum/1
  mod (pu)/1 -> deg2rad1/1
  V7/1 -> V0/2
  V8/1 -> V0/3
  V3/1 -> V0/4
  V0/1 -> Multiport Switch1/4
  choose zero-vector/1(zv) -> V0/1

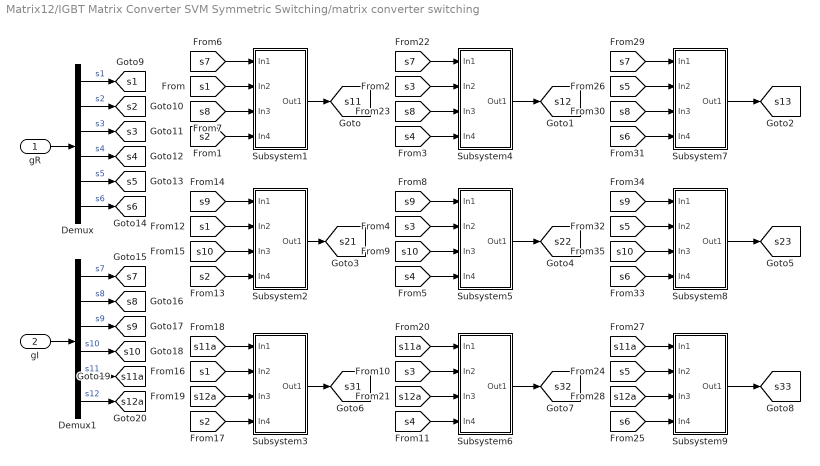
== system Matrix12/IGBT Matrix Converter SVM Symmetric Switching/matrix converter switching ==
  gR : Inport
  gI : Inport  Port=2
  Demux : Demux  Outputs=6
  Demux1 : Demux  Outputs=6
  Subsystem1 : Subsystem
  Subsystem2 : Subsystem
  Subsystem3 : Subsystem
  Subsystem4 : Subsystem
  Subsystem5 : Subsystem
  Subsystem6 : Subsystem
  Subsystem7 : Subsystem
  Subsystem8 : Subsystem
  Subsystem9 : Subsystem
  tag scope: s10=global, s11=global, s11a=global, s12=global, s12a=global, s13=global, s1=global, s21=global, s22=global, s23=global, s2=global, s31=global, s32=global, s33=global, s3=global, s4=global, s5=global, s6=global, s7=global, s8=global, s9=global
  wires:
  Demux/4 -> [s4]  "s4"
  Demux1/6 -> [s12a]  "s12"
  gR/1 -> Demux/1
  gI/1 -> Demux1/1
  Demux/1 -> [s1]  "s1"
  Demux1/5 -> [s11a]  "s11"
  Demux1/4 -> [s10]  "s10"
  Demux1/3 -> [s9]  "s9"
  Demux1/2 -> [s8]  "s8"
  Demux1/1 -> [s7]  "s7"
  Demux/2 -> [s2]  "s2"
  Demux/3 -> [s3]  "s3"
  Demux/5 -> [s5]  "s5"
  Demux/6 -> [s6]  "s6"
  [s7] -> Subsystem1/1(In1)
  [s1] -> Subsystem1/2(In2)
  [s8] -> Subsystem1/3(In3)
  [s2] -> Subsystem1/4(In4)
  [s9] -> Subsystem2/1(In1)
  [s1] -> Subsystem2/2(In2)
  [s10] -> Subsystem2/3(In3)
  [s2] -> Subsystem2/4(In4)
  [s11a] -> Subsystem3/1(In1)
  [s1] -> Subsystem3/2(In2)
  [s12a] -> Subsystem3/3(In3)
  [s2] -> Subsystem3/4(In4)
  [s7] -> Subsystem4/1(In1)
  [s3] -> Subsystem4/2(In2)
  [s8] -> Subsystem4/3(In3)
  [s4] -> Subsystem4/4(In4)
  [s9] -> Subsystem5/1(In1)
  [s3] -> Subsystem5/2(In2)
  [s10] -> Subsystem5/3(In3)
  [s4] -> Subsystem5/4(In4)
  [s11a] -> Subsystem6/1(In1)
  [s3] -> Subsystem6/2(In2)
  [s12a] -> Subsystem6/3(In3)
  [s4] -> Subsystem6/4(In4)
  [s7] -> Subsystem7/1(In1)
  [s5] -> Subsystem7/2(In2)
  [s8] -> Subsystem7/3(In3)
  [s6] -> Subsystem7/4(In4)
  [s9] -> Subsystem8/1(In1)
  [s5] -> Subsystem8/2(In2)
  [s10] -> Subsystem8/3(In3)
  [s6] -> Subsystem8/4(In4)
  [s11a] -> Subsystem9/1(In1)
  [s5] -> Subsystem9/2(In2)
  [s12a] -> Subsystem9/3(In3)
  [s6] -> Subsystem9/4(In4)
  Subsystem1/1(Out1) -> [s11]
  Subsystem4/1(Out1) -> [s12]
  Subsystem7/1(Out1) -> [s13]
  Subsystem2/1(Out1) -> [s21]
  Subsystem5/1(Out1) -> [s22]
  Subsystem8/1(Out1) -> [s23]
  Subsystem3/1(Out1) -> [s31]
  Subsystem6/1(Out1) -> [s32]
  Subsystem9/1(Out1) -> [s33]

== system Matrix12/Matrix Converter/S1 ==
  g : Inport
  Diode : spsDiodeLib/Diode  Ron=0.001  Lon=0  Vf=0  IC=0  UseSnubber=off  Rs=1e4  Cs=250e-9  Measurements=off
  Diode1 : spsDiodeLib/Diode  Ron=0.001  Lon=0  Vf=0  IC=0  UseSnubber=off  Rs=1e4  Cs=250e-9  Measurements=off
  IGBT1 : spsIGBTLib/IGBT  Ron=0.001  Lon=0  Vf=1  Tf=1e-6  Tt=2e-6  IC=0  Rs=1e5  Cs=inf  Measurements=off
  IGBT2 : spsIGBTLib/IGBT  Ron=0.001  Lon=0  Vf=1  Tf=1e-6  Tt=2e-6  IC=0  Rs=1e5  Cs=inf  Measurements=off
  + : PMIOPort  Side=Left
  - : PMIOPort  Port=2  Side=Right
  wires:
  g/1 -> IGBT2/1, IGBT1/1
  connections:
  IGBT2/LConn1 -- Diode/RConn1 -- +/RConn1
  IGBT1/LConn1 -- Diode1/RConn1 -- -/RConn1
  IGBT2/RConn1 -- IGBT1/RConn1 -- Diode/LConn1 -- Diode1/LConn1

== system Matrix12/Matrix Converter/S2 ==
  g : Inport
  Diode : spsDiodeLib/Diode  Ron=0.001  Lon=0  Vf=0  IC=0  UseSnubber=off  Rs=1e4  Cs=250e-9  Measurements=off
  Diode1 : spsDiodeLib/Diode  Ron=0.001  Lon=0  Vf=0  IC=0  UseSnubber=off  Rs=1e4  Cs=250e-9  Measurements=off
  IGBT1 : spsIGBTLib/IGBT  Ron=0.001  Lon=0  Vf=1  Tf=1e-6  Tt=2e-6  IC=0  Rs=1e5  Cs=inf  Measurements=off
  IGBT2 : spsIGBTLib/IGBT  Ron=0.001  Lon=0  Vf=1  Tf=1e-6  Tt=2e-6  IC=0  Rs=1e5  Cs=inf  Measurements=off
  + : PMIOPort  Side=Left
  - : PMIOPort  Port=2  Side=Right
  wires:
  g/1 -> IGBT1/1, IGBT2/1
  connections:
  Diode1/LConn1 -- IGBT1/RConn1 -- IGBT2/RConn1 -- Diode/LConn1
  Diode1/RConn1 -- IGBT1/LConn1 -- -/RConn1
  Diode/RConn1 -- IGBT2/LConn1 -- +/RConn1

== system Matrix12/Matrix Converter/S3 ==
  g : Inport
  Diode : spsDiodeLib/Diode  Ron=0.001  Lon=0  Vf=0  IC=0  UseSnubber=off  Rs=1e4  Cs=250e-9  Measurements=off
  Diode1 : spsDiodeLib/Diode  Ron=0.001  Lon=0  Vf=0  IC=0  UseSnubber=off  Rs=1e4  Cs=250e-9  Measurements=off
  IGBT1 : spsIGBTLib/IGBT  Ron=0.001  Lon=0  Vf=1  Tf=1e-6  Tt=2e-6  IC=0  Rs=1e5  Cs=inf  Measurements=off
  IGBT2 : spsIGBTLib/IGBT  Ron=0.001  Lon=0  Vf=1  Tf=1e-6  Tt=2e-6  IC=0  Rs=1e5  Cs=inf  Measurements=off
  + : PMIOPort  Side=Left
  - : PMIOPort  Port=2  Side=Right
  wires:
  g/1 -> IGBT2/1, IGBT1/1
  connections:
  +/RConn1 -- IGBT2/LConn1 -- Diode/RConn1
  -/RConn1 -- IGBT1/LConn1 -- Diode1/RConn1
  Diode/LConn1 -- IGBT2/RConn1 -- IGBT1/RConn1 -- Diode1/LConn1

== system Matrix12/Matrix Converter/S4 ==
  g : Inport
  Diode : spsDiodeLib/Diode  Ron=0.001  Lon=0  Vf=0  IC=0  UseSnubber=off  Rs=1e4  Cs=250e-9  Measurements=off
  Diode1 : spsDiodeLib/Diode  Ron=0.001  Lon=0  Vf=0  IC=0  UseSnubber=off  Rs=1e4  Cs=250e-9  Measurements=off
  IGBT1 : spsIGBTLib/IGBT  Ron=0.001  Lon=0  Vf=1  Tf=1e-6  Tt=2e-6  IC=0  Rs=1e5  Cs=inf  Measurements=off
  IGBT2 : spsIGBTLib/IGBT  Ron=0.001  Lon=0  Vf=1  Tf=1e-6  Tt=2e-6  IC=0  Rs=1e5  Cs=inf  Measurements=off
  + : PMIOPort  Side=Left
  - : PMIOPort  Port=2  Side=Right
  wires:
  g/1 -> IGBT1/1, IGBT2/1
  connections:
  Diode1/LConn1 -- IGBT1/RConn1 -- IGBT2/RConn1 -- Diode/LConn1
  Diode1/RConn1 -- IGBT1/LConn1 -- -/RConn1
  Diode/RConn1 -- IGBT2/LConn1 -- +/RConn1

== system Matrix12/Matrix Converter/S5 ==
  g : Inport
  Diode : spsDiodeLib/Diode  Ron=0.001  Lon=0  Vf=0  IC=0  UseSnubber=off  Rs=1e4  Cs=250e-9  Measurements=off
  Diode1 : spsDiodeLib/Diode  Ron=0.001  Lon=0  Vf=0  IC=0  UseSnubber=off  Rs=1e4  Cs=250e-9  Measurements=off
  IGBT1 : spsIGBTLib/IGBT  Ron=0.001  Lon=0  Vf=1  Tf=1e-6  Tt=2e-6  IC=0  Rs=1e5  Cs=inf  Measurements=off
  IGBT2 : spsIGBTLib/IGBT  Ron=0.001  Lon=0  Vf=1  Tf=1e-6  Tt=2e-6  IC=0  Rs=1e5  Cs=inf  Measurements=off
  + : PMIOPort  Side=Left
  - : PMIOPort  Port=2  Side=Right
  wires:
  g/1 -> IGBT2/1, IGBT1/1
  connections:
  +/RConn1 -- IGBT2/LConn1 -- Diode/RConn1
  -/RConn1 -- IGBT1/LConn1 -- Diode1/RConn1
  Diode/LConn1 -- IGBT2/RConn1 -- IGBT1/RConn1 -- Diode1/LConn1

== system Matrix12/Matrix Converter/S6 ==
  g : Inport
  Diode : spsDiodeLib/Diode  Ron=0.001  Lon=0  Vf=0  IC=0  UseSnubber=off  Rs=1e4  Cs=250e-9  Measurements=off
  Diode1 : spsDiodeLib/Diode  Ron=0.001  Lon=0  Vf=0  IC=0  UseSnubber=off  Rs=1e4  Cs=250e-9  Measurements=off
  IGBT1 : spsIGBTLib/IGBT  Ron=0.001  Lon=0  Vf=1  Tf=1e-6  Tt=2e-6  IC=0  Rs=1e5  Cs=inf  Measurements=off
  IGBT2 : spsIGBTLib/IGBT  Ron=0.001  Lon=0  Vf=1  Tf=1e-6  Tt=2e-6  IC=0  Rs=1e5  Cs=inf  Measurements=off
  + : PMIOPort  Side=Left
  - : PMIOPort  Port=2  Side=Right
  wires:
  g/1 -> IGBT1/1, IGBT2/1
  connections:
  Diode1/LConn1 -- IGBT1/RConn1 -- IGBT2/RConn1 -- Diode/LConn1
  Diode1/RConn1 -- IGBT1/LConn1 -- -/RConn1
  Diode/RConn1 -- IGBT2/LConn1 -- +/RConn1

== system Matrix12/Matrix Converter/S7 ==
  g : Inport
  Diode : spsDiodeLib/Diode  Ron=0.001  Lon=0  Vf=0  IC=0  UseSnubber=off  Rs=1e4  Cs=250e-9  Measurements=off
  Diode1 : spsDiodeLib/Diode  Ron=0.001  Lon=0  Vf=0  IC=0  UseSnubber=off  Rs=1e4  Cs=250e-9  Measurements=off
  IGBT1 : spsIGBTLib/IGBT  Ron=0.001  Lon=0  Vf=1  Tf=1e-6  Tt=2e-6  IC=0  Rs=1e5  Cs=inf  Measurements=off
  IGBT2 : spsIGBTLib/IGBT  Ron=0.001  Lon=0  Vf=1  Tf=1e-6  Tt=2e-6  IC=0  Rs=1e5  Cs=inf  Measurements=off
  + : PMIOPort  Side=Left
  - : PMIOPort  Port=2  Side=Right
  wires:
  g/1 -> IGBT2/1, IGBT1/1
  connections:
  +/RConn1 -- IGBT2/LConn1 -- Diode/RConn1
  -/RConn1 -- IGBT1/LConn1 -- Diode1/RConn1
  Diode/LConn1 -- IGBT2/RConn1 -- IGBT1/RConn1 -- Diode1/LConn1

== system Matrix12/Matrix Converter/S8 ==
  g : Inport
  Diode : spsDiodeLib/Diode  Ron=0.001  Lon=0  Vf=0  IC=0  UseSnubber=off  Rs=1e4  Cs=250e-9  Measurements=off
  Diode1 : spsDiodeLib/Diode  Ron=0.001  Lon=0  Vf=0  IC=0  UseSnubber=off  Rs=1e4  Cs=250e-9  Measurements=off
  IGBT1 : spsIGBTLib/IGBT  Ron=0.001  Lon=0  Vf=1  Tf=1e-6  Tt=2e-6  IC=0  Rs=1e5  Cs=inf  Measurements=off
  IGBT2 : spsIGBTLib/IGBT  Ron=0.001  Lon=0  Vf=1  Tf=1e-6  Tt=2e-6  IC=0  Rs=1e5  Cs=inf  Measurements=off
  + : PMIOPort  Side=Left
  - : PMIOPort  Port=2  Side=Right
  wires:
  g/1 -> IGBT1/1, IGBT2/1
  connections:
  Diode1/LConn1 -- IGBT1/RConn1 -- IGBT2/RConn1 -- Diode/LConn1
  Diode1/RConn1 -- IGBT1/LConn1 -- -/RConn1
  Diode/RConn1 -- IGBT2/LConn1 -- +/RConn1

== system Matrix12/Matrix Converter/S9 ==
  g : Inport
  Diode : spsDiodeLib/Diode  Ron=0.001  Lon=0  Vf=0  IC=0  UseSnubber=off  Rs=1e4  Cs=250e-9  Measurements=off
  Diode1 : spsDiodeLib/Diode  Ron=0.001  Lon=0  Vf=0  IC=0  UseSnubber=off  Rs=1e4  Cs=250e-9  Measurements=off
  IGBT1 : spsIGBTLib/IGBT  Ron=0.001  Lon=0  Vf=1  Tf=1e-6  Tt=2e-6  IC=0  Rs=1e5  Cs=inf  Measurements=off
  IGBT2 : spsIGBTLib/IGBT  Ron=0.001  Lon=0  Vf=1  Tf=1e-6  Tt=2e-6  IC=0  Rs=1e5  Cs=inf  Measurements=off
  + : PMIOPort  Side=Left
  - : PMIOPort  Port=2  Side=Right
  wires:
  g/1 -> IGBT2/1, IGBT1/1
  connections:
  +/RConn1 -- IGBT2/LConn1 -- Diode/RConn1
  -/RConn1 -- IGBT1/LConn1 -- Diode1/RConn1
  Diode/LConn1 -- IGBT2/RConn1 -- IGBT1/RConn1 -- Diode1/LConn1

== system Matrix12/Shunt Active Filter/Subsystem3 ==
  pb : Inport
  Valpha : Inport  Port=2
  "Vbeta " : Inport  Port=3
  qb : Inport  Port=4
  Add : Sum
  Add1 : Sum  Inputs=+-
  Fcn : Fcn  Expr=1/(u(1)^2+u(2)^2)
  Mux : Mux  Inputs=2
  Product{,1..5} (6 alike) : Product
  i*alpha : Outport  VectorParamsAs1DForOutWhenUnconnected=off
  "I*beta " : Outport  Port=2  VectorParamsAs1DForOutWhenUnconnected=off
  wires:
  Product1/1 -> Add/2
  Product2/1 -> Add1/1
  pb/1 -> Product2/1, Product/1
  Product4/1 -> i*alpha/1
  Fcn/1 -> Product5/2, Product4/2
  "Vbeta "/1 -> Mux/2, Product2/2, Product1/2
  Product3/1 -> Add1/2
  Valpha/1 -> Mux/1, Product3/2, Product/2
  qb/1 -> Product1/1, Product3/1
  Add/1 -> Product4/1
  Mux/1 -> Fcn/1
  Product/1 -> Add/1
  Add1/1 -> Product5/1
  Product5/1 -> "I*beta "/1

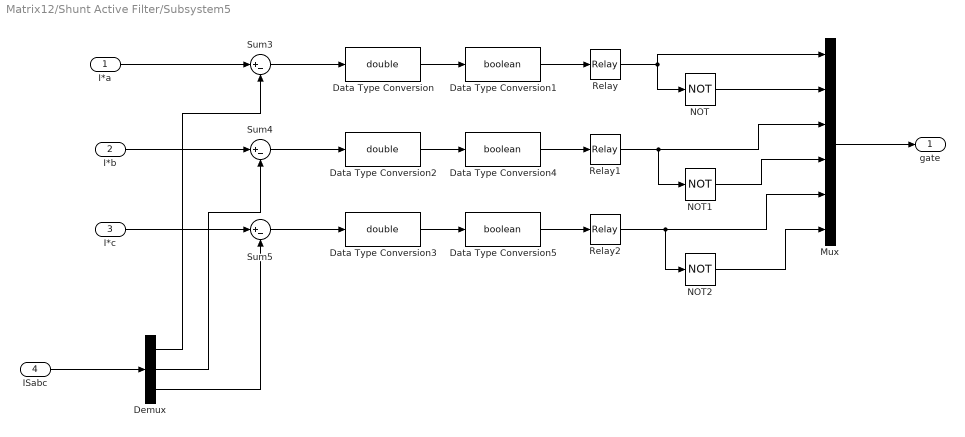
== system Matrix12/Shunt Active Filter/Subsystem5 ==
  I*a : Inport
  I*b : Inport  Port=2
  I*c : Inport  Port=3
  ISabc : Inport  Port=4
  Data Type Conversion : DataTypeConversion  OutDataTypeStr=double
  Data Type Conversion1 : DataTypeConversion  OutDataTypeStr=boolean
  Data Type Conversion2 : DataTypeConversion  OutDataTypeStr=double
  Data Type Conversion3 : DataTypeConversion  OutDataTypeStr=double
  Data Type Conversion4 : DataTypeConversion  OutDataTypeStr=boolean
  Data Type Conversion5 : DataTypeConversion  OutDataTypeStr=boolean
  Demux : Demux  Outputs=3
  Mux : Mux  Inputs=6
  NOT : Logic  Operator=NOT  AllPortsSameDT=off  OutDataTypeStr=boolean
  NOT1 : Logic  Operator=NOT  AllPortsSameDT=off  OutDataTypeStr=boolean
  NOT2 : Logic  Operator=NOT  AllPortsSameDT=off  OutDataTypeStr=boolean
  Relay : Relay  OnSwitchValue=1  OffSwitchValue=0
  Relay1 : Relay  OnSwitchValue=1  OffSwitchValue=0
  Relay2 : Relay  OnSwitchValue=1  OffSwitchValue=0
  Sum3 : Sum  Inputs=|+-
  Sum4 : Sum  Inputs=|+-
  Sum5 : Sum  Inputs=|+-
  "gate " : Outport  VectorParamsAs1DForOutWhenUnconnected=off
  wires:
  Data Type Conversion/1 -> Data Type Conversion1/1
  I*a/1 -> Sum3/1
  Mux/1 -> "gate "/1
  Demux/2 -> Sum4/2
  ISabc/1 -> Demux/1
  Data Type Conversion5/1 -> Relay2/1
  Sum5/1 -> Data Type Conversion3/1
  Relay2/1 -> NOT2/1, Mux/5
  Relay1/1 -> NOT1/1, Mux/3
  NOT1/1 -> Mux/4
  NOT2/1 -> Mux/6
  Data Type Conversion4/1 -> Relay1/1
  Data Type Conversion1/1 -> Relay/1
  NOT/1 -> Mux/2
  Relay/1 -> NOT/1, Mux/1
  Data Type Conversion3/1 -> Data Type Conversion5/1
  I*c/1 -> Sum5/1
  Sum3/1 -> Data Type Conversion/1
  Sum4/1 -> Data Type Conversion2/1
  Data Type Conversion2/1 -> Data Type Conversion4/1
  Demux/1 -> Sum3/2
  Demux/3 -> Sum5/2
  I*b/1 -> Sum4/1

== system Matrix12/Shunt Active Filter/pq ==
  Valpha : Inport
  Vbeta : Inport  Port=2
  Ialpha : Inport  Port=3
  Ibeta : Inport  Port=4
  Product{,1..3} (4 alike) : Product
  Sum : Sum
  Sum1 : Sum  Inputs=+-
  P : Outport  VectorParamsAs1DForOutWhenUnconnected=off
  Q : Outport  Port=2  VectorParamsAs1DForOutWhenUnconnected=off
  wires:
  Product2/1 -> Sum1/1
  Ialpha/1 -> Product2/1, Product/2
  Ibeta/1 -> Product1/2, Product3/1
  Vbeta/1 -> Product2/2, Product1/1
  Product1/1 -> Sum/2
  Valpha/1 -> Product3/2, Product/1
  Sum/1 -> P/1
  Product3/1 -> Sum1/2
  Product/1 -> Sum/1
  Sum1/1 -> Q/1

== system Matrix12/IGBT Matrix Converter SVM Symmetric Switching/SVM Inversion symmetric sequence/Calculate duty-cycles ==
  deg_mag : Inport
  Trigger : TriggerPort  VariantControl=Variant
  Constant : Constant  Value=pi/3
  Constant1 : Constant
  Demux : Demux  Outputs=2
  Mux : Mux  Inputs=2
  Mux1 : Mux  Inputs=2
  Product : Product  Inputs=**  RndMeth=Zero
  Sum : Sum  Inputs=+-
  Sum of Elements : Sum  Inputs=+
  Sum1 : Sum  Inputs=-+
  Sum2 : Sum  Inputs=-+
  Trigonometric Function : Trigonometry  Operator=cos
  Trigonometric Function1 : Trigonometry
  deg2rad : Gain  Gain=pi/180
  deg2rad1 : Gain  Gain=0.5/0.866
  d1_d2_d0 : Outport  VectorParamsAs1DForOutWhenUnconnected=off
  wires:
  Sum of Elements/1 -> Sum2/1
  Constant1/1 -> Sum2/2
  Sum2/1 -> Mux1/2  "d0"
  Mux1/1 -> d1_d2_d0/1
  Product/1 -> Sum of Elements/1, Mux1/1  "d1 d2"
  Constant/1 -> Sum1/2
  Mux/1 -> Trigonometric Function1/1, Trigonometric Function/1
  Sum1/1 -> Mux/2
  deg2rad/1 -> Sum1/1, Mux/1  "theta"
  Sum/1 -> Product/1
  Trigonometric Function1/1 -> deg2rad1/1
  Trigonometric Function/1 -> Sum/1
  Demux/2 -> Product/2  "mag"
  Demux/1 -> deg2rad/1
  deg_mag/1 -> Demux/1
  deg2rad1/1 -> Sum/2

== system Matrix12/IGBT Matrix Converter SVM Symmetric Switching/SVM Inversion symmetric sequence/Triggered Subsystem ==
  In1 : Inport
  Trigger : TriggerPort  VariantControl=Variant
  Out1 : Outport  VectorParamsAs1DForOutWhenUnconnected=off
  wires:
  In1/1 -> Out1/1

== system Matrix12/IGBT Matrix Converter SVM Symmetric Switching/SVM Inversion symmetric sequence/abc 2 alpha-beta ==
  Vabc : Inport
  Demux : Demux  Outputs=3
      settings: DisplayOption=none
  Gain : Gain  Gain=1/2  SaturateOnIntegerOverflow=on  OutDataTypeStr=Inherit: Same as input  ParamDataTypeStr=Inherit: Same as input
  Gain1 : Gain  Gain=1/2  SaturateOnIntegerOverflow=on  OutDataTypeStr=Inherit: Same as input  ParamDataTypeStr=Inherit: Same as input
  Gain2 : Gain  Gain=sqrt(2/3)  SaturateOnIntegerOverflow=on  OutDataTypeStr=Inherit: Same as input  ParamDataTypeStr=Inherit: Same as input
  Gain3 : Gain  Gain=sqrt(3)/2  SaturateOnIntegerOverflow=on  OutDataTypeStr=Inherit: Same as input  ParamDataTypeStr=Inherit: Same as input
  Gain4 : Gain  Gain=sqrt(3)/2  SaturateOnIntegerOverflow=on  OutDataTypeStr=Inherit: Same as input  ParamDataTypeStr=Inherit: Same as input
  Gain5 : Gain  Gain=sqrt(2/3)  SaturateOnIntegerOverflow=on  OutDataTypeStr=Inherit: Same as input  ParamDataTypeStr=Inherit: Same as input
  Sum : Sum  Inputs=+--  InputSameDT=on  SaturateOnIntegerOverflow=on  OutDataTypeStr=Inherit: Same as first input
  Sum1 : Sum  Inputs=+-  InputSameDT=on  SaturateOnIntegerOverflow=on  OutDataTypeStr=Inherit: Same as first input
  Valpha : Outport  VectorParamsAs1DForOutWhenUnconnected=off
  Vbeta : Outport  Port=2  VectorParamsAs1DForOutWhenUnconnected=off
  wires:
  Gain5/1 -> Vbeta/1
  Gain2/1 -> Valpha/1
  Vabc/1 -> Demux/1
  Gain3/1 -> Sum1/1
  Gain4/1 -> Sum1/2
  Sum1/1 -> Gain5/1
  Sum/1 -> Gain2/1
  Gain1/1 -> Sum/3
  Gain/1 -> Sum/2
  Demux/1 -> Sum/1
  Demux/2 -> Gain/1, Gain3/1
  Demux/3 -> Gain1/1, Gain4/1

== system Matrix12/IGBT Matrix Converter SVM Symmetric Switching/SVM Inversion symmetric sequence/alpha-beta 2 deg-mag ==
  Valpha : Inport
  Vbeta : Inport  Port=2
  Math Function : Math  Operator=square  SignedPower=on  SaturateOnIntegerOverflow=on
  Math Function1 : Math  Operator=sqrt  SignedPower=on  SaturateOnIntegerOverflow=on
  Mux1 : Mux  Inputs=2
  Sum of Elements : Sum  Inputs=+
  Trigonometric Function : Trigonometry  Operator=atan2
  rad2deg : Gain  Gain=180/pi  SaturateOnIntegerOverflow=on  OutDataTypeStr=Inherit: Same as input  ParamDataTypeStr=Inherit: Same as input
  Vdeg : Outport  VectorParamsAs1DForOutWhenUnconnected=off
  Vmag : Outport  Port=2  VectorParamsAs1DForOutWhenUnconnected=off
  wires:
  Math Function1/1 -> Vmag/1
  rad2deg/1 -> Vdeg/1
  Vbeta/1 -> Mux1/2, Trigonometric Function/1
  Sum of Elements/1 -> Math Function1/1
  Math Function/1 -> Sum of Elements/1
  Mux1/1 -> Math Function/1
  Valpha/1 -> Mux1/1, Trigonometric Function/2
  Trigonometric Function/1 -> rad2deg/1

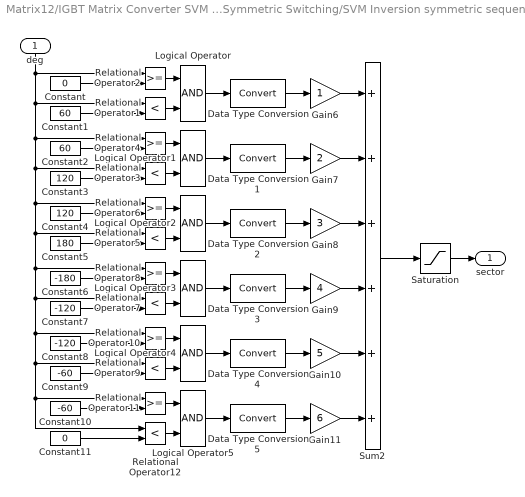
== system Matrix12/IGBT Matrix Converter SVM Symmetric Switching/SVM Inversion symmetric sequence/sector ==
  deg : Inport
  Constant : Constant  Value=0
  Constant1 : Constant  Value=60
  Constant10 : Constant  Value=-60
  Constant11 : Constant  Value=0
  Constant2 : Constant  Value=60
  Constant3 : Constant  Value=120
  Constant4 : Constant  Value=120
  Constant5 : Constant  Value=180
  Constant6 : Constant  Value=-180
  Constant7 : Constant  Value=-120
  Constant8 : Constant  Value=-120
  Constant9 : Constant  Value=-60
  Data Type Conversion{,1..5} (6 alike) : DataTypeConversion  SaturateOnIntegerOverflow=on  RndMeth=Zero
  Gain10 : Gain  Gain=5  SaturateOnIntegerOverflow=on  OutDataTypeStr=Inherit: Same as input  ParamDataTypeStr=Inherit: Same as input
  Gain11 : Gain  Gain=6  SaturateOnIntegerOverflow=on  OutDataTypeStr=Inherit: Same as input  ParamDataTypeStr=Inherit: Same as input
  Gain6 : Gain  SaturateOnIntegerOverflow=on  OutDataTypeStr=Inherit: Same as input  ParamDataTypeStr=Inherit: Same as input
  Gain7 : Gain  Gain=2  SaturateOnIntegerOverflow=on  OutDataTypeStr=Inherit: Same as input  ParamDataTypeStr=Inherit: Same as input
  Gain8 : Gain  Gain=3  SaturateOnIntegerOverflow=on  OutDataTypeStr=Inherit: Same as input  ParamDataTypeStr=Inherit: Same as input
  Gain9 : Gain  Gain=4  SaturateOnIntegerOverflow=on  OutDataTypeStr=Inherit: Same as input  ParamDataTypeStr=Inherit: Same as input
  Logical Operator{,1..5} (6 alike) : Logic
  Relational Operator{1,3,5,7,9,12} (6 alike) : RelationalOperator  Operator=<  RndMeth=Nearest  InputSameDT=on
  Relational Operator{2,4,6,8,10..11} (6 alike) : RelationalOperator  RndMeth=Nearest  InputSameDT=on
  Saturation : Saturate  UpperLimit=6  LowerLimit=1
  Sum2 : Sum  Inputs=++++++  InputSameDT=on  SaturateOnIntegerOverflow=on  OutDataTypeStr=Inherit: Same as first input
  sector : Outport  VectorParamsAs1DForOutWhenUnconnected=off
  wires:
  Saturation/1 -> sector/1
  deg/1 -> Relational Operator2/1, Relational Operator1/1, Relational Operator4/1, Relational Operator3/1, Relational Operator6/1, Relational Operator5/1, Relational Operator8/1, Relational Operator7/1, Relational Operator10/1, Relational Operator9/1, Relational Operator11/1, Relational Operator12/1
  Data Type Conversion5/1 -> Gain11/1
  Data Type Conversion4/1 -> Gain10/1
  Data Type Conversion3/1 -> Gain9/1
  Data Type Conversion2/1 -> Gain8/1
  Data Type Conversion1/1 -> Gain7/1
  Data Type Conversion/1 -> Gain6/1
  Relational Operator2/1 -> Logical Operator/1
  Relational Operator1/1 -> Logical Operator/2
  Logical Operator/1 -> Data Type Conversion/1
  Constant/1 -> Relational Operator2/2
  Constant1/1 -> Relational Operator1/2
  Relational Operator4/1 -> Logical Operator1/1
  Relational Operator3/1 -> Logical Operator1/2
  Logical Operator1/1 -> Data Type Conversion1/1
  Constant2/1 -> Relational Operator4/2
  Constant3/1 -> Relational Operator3/2
  Relational Operator6/1 -> Logical Operator2/1
  Relational Operator5/1 -> Logical Operator2/2
  Logical Operator2/1 -> Data Type Conversion2/1
  Constant4/1 -> Relational Operator6/2
  Constant5/1 -> Relational Operator5/2
  Relational Operator8/1 -> Logical Operator3/1
  Relational Operator7/1 -> Logical Operator3/2
  Logical Operator3/1 -> Data Type Conversion3/1
  Constant6/1 -> Relational Operator8/2
  Constant7/1 -> Relational Operator7/2
  Relational Operator10/1 -> Logical Operator4/1
  Relational Operator9/1 -> Logical Operator4/2
  Logical Operator4/1 -> Data Type Conversion4/1
  Constant8/1 -> Relational Operator10/2
  Constant9/1 -> Relational Operator9/2
  Relational Operator11/1 -> Logical Operator5/1
  Relational Operator12/1 -> Logical Operator5/2
  Logical Operator5/1 -> Data Type Conversion5/1
  Constant10/1 -> Relational Operator11/2
  Constant11/1 -> Relational Operator12/2
  Gain6/1 -> Sum2/1
  Gain7/1 -> Sum2/2
  Gain8/1 -> Sum2/3
  Gain9/1 -> Sum2/4
  Gain10/1 -> Sum2/5
  Gain11/1 -> Sum2/6
  Sum2/1 -> Saturation/1
